simulink model "satmodel"  (R2023b)
settings: Solver=FixedStepAuto  StartTime=0.0  StopTime=5000  FixedStep=0.01  MaxStep=1  RelTol=1e-6  EnableMultiTasking=on
undefined symbols (not defined in the file or in its folder): A, C, CtransW
settings Model: Creator=Scott.Dahlke  LastModifiedBy=Connor Emmons
settings SolverCC: AlgebraicLoopSolver=TrustRegion
settings DataIOCC: LimitDataPoints=on  MaxDataPoints=10000  SaveFormat=Array  SignalLoggingSaveFormat=ModelDataLogs  ReturnWorkspaceOutputs=off
settings OptimizationCC: ExpressionDepthLimit=2147483647  InitFltsAndDblsToZero=on  LifeSpan=inf
settings DebuggingCC: UnderspecifiedInitializationDetection=Classic  MergeDetectMultiDrivingBlocksExec=none  SolverPrmCheckMsg=warning  FcnCallInpInsideContextMsg=warning  UnconnectedInputMsg=warning  UnconnectedOutputMsg=warning  UnconnectedLineMsg=warning  StateNameClashWarn=warning  SFUnexpectedBacktrackingDiag=warning  SFNoUnconditionalDefaultTransitionDiag=warning  SFExecutionAtInitializationDiag=none  ArithmeticOperatorsInVariantConditions=warning
settings HardwareCC: ProdBitPerPointer=32  ProdBitPerSizeT=32  ProdBitPerPtrDiffT=32  ProdLargestAtomicFloat=None  ProdIntDivRoundTo=Undefined  ProdEndianess=Unspecified  ProdWordSize=32  ProdHWDeviceType=32-bit Generic
settings ModelReferenceCC: EnableRefExpFcnMdlSchedulingChecks=on  PropagateSignalLabelsOutOfModel=off
settings CodeAppCC: StateflowObjectComments=on
settings GRTTargetCC: TargetLangStandard=C89/C90 (ANSI)  CombineOutputUpdateFcns=off  GRTInterface=on
settings ConfigComp: CovMetricSettings=dw  CovSaveCumulativeToWorkspaceVar=on  CovSaveSingleToWorkspaceVar=on

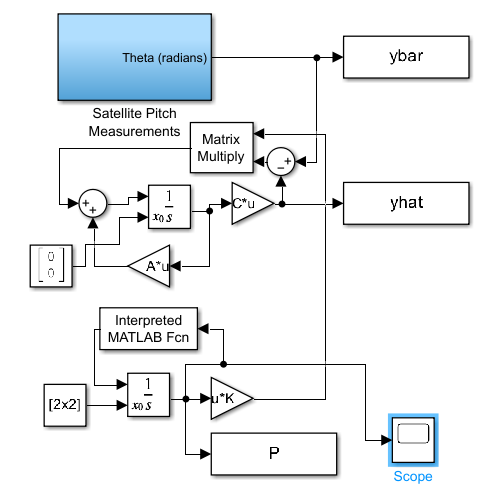
[thumbnail: Simulink's stored preview of the top-level diagram]
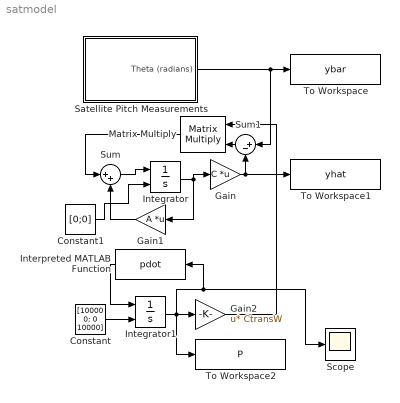
== system satmodel ==
  Constant : Constant  Value=[10000 0; 0 10000]  VectorParams1D=off
  Constant1 : Constant  Value=[0;0]  VectorParams1D=off
  Gain : Gain  Gain=C  Multiplication=Matrix(K*u)
  Gain1 : Gain  Gain=A  Multiplication=Matrix(K*u)
  Gain2 : Gain  Gain=CtransW  Multiplication=Matrix(u*K)
  Integrator : Integrator  InitialConditionSource=external
  Integrator1 : Integrator  InitialConditionSource=external
  Interpreted MATLAB Function : MATLABFcn  MATLABFcn=pdot  Output1D=off
  Matrix Multiply : Product  Multiplication=Matrix(*)
  Satellite Pitch Measurements : Subsystem
  Scope : Scope
  Sum : Sum  Inputs=|++
  Sum1 : Sum  Inputs=|+-
  To Workspace : ToWorkspace  VariableName=ybar  SampleTime=-1
  To Workspace1 : ToWorkspace  VariableName=yhat  SampleTime=-1
      settings: Save2DSignal=2-D array (concatenate along first dimension)
  To Workspace2 : ToWorkspace  VariableName=P  SampleTime=-1
      settings: Save2DSignal=2-D array (concatenate along first dimension)
  wires:
  Satellite Pitch Measurements/1(Theta (radians)) -> Sum1/1, To Workspace/1
  Sum/1 -> Integrator/1
  Integrator/1 -> Gain/1, Gain1/1
  Gain1/1 -> Sum/2
  Gain/1 -> To Workspace1/1, Sum1/2
  Integrator1/1 -> Scope/1, Interpreted MATLAB Function/1, To Workspace2/1, Gain2/1
  Constant/1 -> Integrator1/2
  Interpreted MATLAB Function/1 -> Integrator1/1
  Sum1/1 -> Matrix Multiply/2
  Gain2/1 -> Matrix Multiply/1
  Matrix Multiply/1 -> Sum/1
  Constant1/1 -> Integrator/2

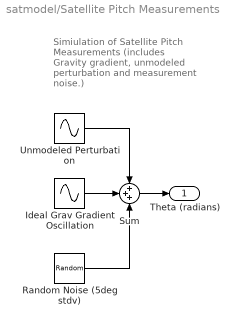
== system satmodel/Satellite Pitch Measurements ==
  note: Simiulation of Satellite
      | Pitch Measurements
      | (includes Gravity gradient,
      | unmodeled perturbation and
      | measurement noise.)
  Ideal Grav Gradient Oscillation : Sin  Amplitude=60*pi/180  Frequency=0.001873018811298  SampleTime=0
  Random Noise (5deg stdv) : RandomNumber  Variance=(5*pi/180)^2  SampleTime=0
  Sum : Sum  Inputs=+++
  Unmodeled Perturbation : Sin  Amplitude=50*pi/180  Frequency=2e-4  SampleTime=0
  Theta (radians) : Outport
  wires:
  Random Noise (5deg stdv)/1 -> Sum/3
  Ideal Grav Gradient Oscillation/1 -> Sum/2
  Unmodeled Perturbation/1 -> Sum/1
  Sum/1 -> Theta (radians)/1
